simulink model "AC_RLC"  (R2022a)
settings: Solver=VariableStepAuto  StartTime=0.0  StopTime=10.0  RelTol=1e-3
model workspace (MAT data in the model file):
  C = 3.5e-06
  L = 0.002
  R = 1230
  f = 1000
settings Model: Creator=Adam Ghatta  LastModifiedBy=Adam Ghatta

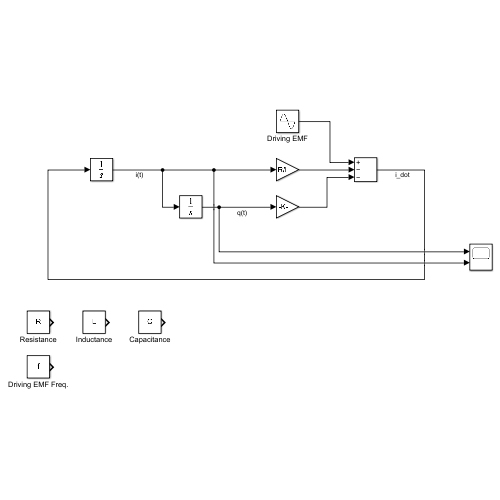
[thumbnail: Simulink's stored preview of the top-level diagram]
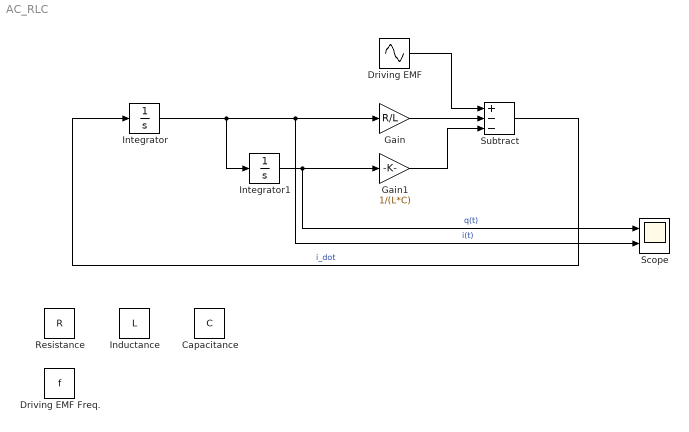
== system AC_RLC ==
  Capacitance : Constant  Value=C
  Driving EMF : Sin  Frequency=2 * pi * f  SampleTime=0
  Driving EMF Freq. : Constant  Value=f
  Gain : Gain  Gain=R/L
  Gain1 : Gain  Gain=1/(L*C)
  Inductance : Constant  Value=L
  Integrator : Integrator
  Integrator1 : Integrator
  Resistance : Constant  Value=R
  Scope : Scope  NumInputPorts=2
  Subtract : Sum  Inputs=+--
  wires:
  Driving EMF/1 -> Subtract/1
  Gain/1 -> Subtract/2
  Gain1/1 -> Subtract/3
  Subtract/1 -> Integrator/1  "i_dot"
  Integrator/1 -> Integrator1/1, Scope/2, Gain/1  "i(t)"
  Integrator1/1 -> Scope/1, Gain1/1  "q(t)"
